simulink model "AOO_Version1"  (R2022a)
settings: Solver=FixedStepAuto  StartTime=0.0  StopTime=inf  FixedStep=1e-3  RelTol=1e-3  EnableMultiTasking=on
undefined symbols (not defined in the file): D10, D11, D12, D2, D4, D5, D7, D8, D9, PTA0, PTA2, PTB23, PTB9, PTC3, PTC4, PTD0, PTD2, PTD3
libraries: frdmk64flib x9
settings Model: ExtModeTrigDuration=5  Creator=ethan  LastModifiedBy=ethan
settings OptimizationCC: EnhancedBackFolding=on  PassReuseOutputArgsAs=Individual arguments  ZeroExternalMemoryAtStartup=off  ZeroInternalMemoryAtStartup=off  MaxStackSize=64  OptimizeBlockOrder=speed  DifferentSizesBufferReuse=on  OptimizationCustomize=off  EfficientTunableParamExpr=on
settings DebuggingCC: ParameterTunabilityLossMsg=error
settings HardwareCC: ProdBitPerPointer=32  ProdBitPerSizeT=32  ProdBitPerPtrDiffT=32  ProdLargestAtomicInteger=Long  ProdLargestAtomicFloat=Double  ProdWordSize=32  ProdHWDeviceType=ARM Compatible->ARM Cortex
settings SFSimCC: MATLABDynamicMemAlloc=off
settings RTWCC: SystemTargetFile=ert.tlc  HardwareBoard=NXP FRDM-K64F  TLCOptions="-aInlineSetEventsForThisBaseRateFcn=TLC_FALSE -aSuppressMultiTaskScheduler=TLC_FALSE  -aRateBasedStepFcn=0"  TemplateMakefile=ert_default_tmf  Toolchain=GNU Tools for ARM Embedded Processors
settings CodeAppCC: ForceParamTrailComments=on  IgnoreCustomStorageClasses=off  OperatorAnnotations=on  SimulinkDataObjDesc=on  SFDataObjDesc=on  InsertBlockDesc=on
settings ERTTargetCC: ExtModeTransport=4  ExtModeMexFile=sendToCommService

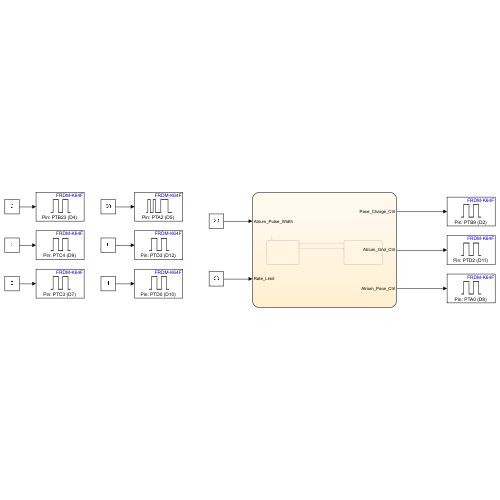
[thumbnail: Simulink's stored preview of the top-level diagram]
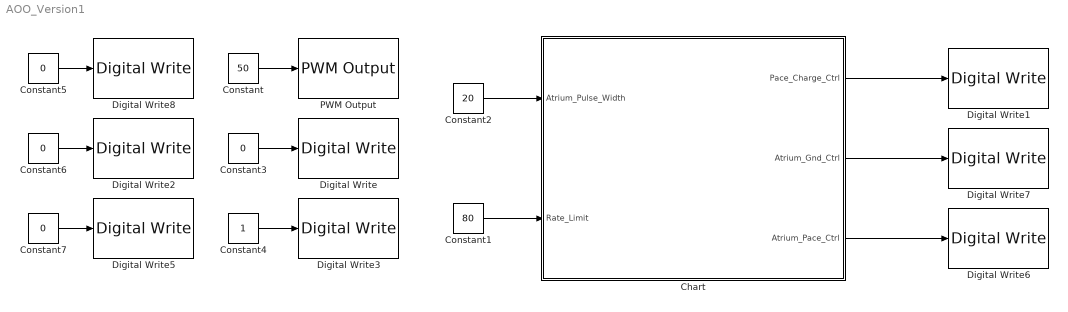
== system AOO_Version1 ==
  Chart : Stateflow chart  TreatAsAtomicUnit=on
  Constant : Constant  Value=50  OutDataTypeStr=int8
  Constant1 : Constant  Value=80  OutDataTypeStr=double
  Constant2 : Constant  Value=20
  Constant{3,5..7} (4 alike) : Constant  Value=0  OutDataTypeStr=int8
  Constant4 : Constant  OutDataTypeStr=int8
  Digital Write : frdmk64flib/Digital Write  Whichpin=PTD3 (D12)
  Digital Write1 : frdmk64flib/Digital Write  Whichpin=PTB9 (D2)
  Digital Write2 : frdmk64flib/Digital Write  Whichpin=PTC4 (D9)
  Digital Write3 : frdmk64flib/Digital Write  Whichpin=PTD0 (D10)
  Digital Write5 : frdmk64flib/Digital Write  Whichpin=PTC3 (D7)
  Digital Write6 : frdmk64flib/Digital Write  Whichpin=PTA0 (D8)
  Digital Write7 : frdmk64flib/Digital Write  Whichpin=PTD2 (D11)
  Digital Write8 : frdmk64flib/Digital Write  Whichpin=PTB23 (D4)
  PWM Output : frdmk64flib/PWM Output  Whichpin=PTA2 (D5)  InitialFrequency=2000  InitialDutyCycle=0
  wires:
  Chart/1(Pace_Charge_Ctrl) -> Digital Write1/1
  Constant1/1 -> Chart/2(Rate_Limit)
  Constant/1 -> PWM Output/1
  Constant2/1 -> Chart/1(Atrium_Pulse_Width)
  Chart/2(Atrium_Gnd_Ctrl) -> Digital Write7/1
  Chart/3(Atrium_Pace_Ctrl) -> Digital Write6/1
  Constant3/1 -> Digital Write/1
  Constant4/1 -> Digital Write3/1
  Constant5/1 -> Digital Write8/1
  Constant6/1 -> Digital Write2/1
  Constant7/1 -> Digital Write5/1

== stateflow chart AOO_Version1/Chart ==
  state Charge_C22
    entry:
    Atrium_Pace_Ctrl = false;
    Atrium_Gnd_Ctrl = true;
    Pace_Charge_Ctrl = true;
  state Discharge_C22
    entry:
    Pace_Charge_Ctrl = false;
    Atrium_Pace_Ctrl = true;
    Atrium_Gnd_Ctrl = false;
  (default) -> Charge_C22
  Discharge_C22 -> Charge_C22 : after(Atrium_Pulse_Width,msec)
  Charge_C22 -> Discharge_C22 : after((60000/Rate_Limit)-Atrium_Pulse_Width,msec)
  data: Pace_Charge_Ctrl output; Atrium_Gnd_Ctrl output; Atrium_Pace_Ctrl output; Atrium_Pulse_Width input; Rate_Limit input
